simulink model "sign"  (Simulink 6.6)
settings: Solver=FixedStepDiscrete  StartTime=0.0  StopTime=10.0  FixedStep=1  RelTol=1e-3
settings Model: Creator=ksmyth  LastModifiedBy=ksmyth

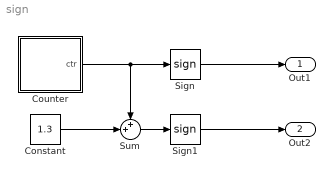
== system sign ==
  Constant : Constant  Value=1.3
  Counter : Stateflow chart
  Sign : Signum
  Sign1 : Signum
  Sum : Sum  Inputs=++|
  Out1 : Outport
  Out2 : Outport  Port=2
  wires:
  Counter/1(ctr) -> Sign/1, Sum/1
  Sign/1 -> Out1/1
  Sum/1 -> Sign1/1
  Sign1/1 -> Out2/1
  Constant/1 -> Sum/2

== stateflow chart Counter ==
  settings: executeAtInitialization=1
  state s1
  (default) -> s1
  s1 -> s1 [order 1] : [ctr < 3] / ctr = ctr+1;
  s1 -> s1 [order 2] : [ctr >= 3] / ctr = -2;
  data: ctr output double =-1
